simulink model "q8"  (R2019a)
settings: Solver=VariableStepAuto  StartTime=0.0  StopTime=2  RelTol=1e-3
libraries: simulink x4
settings Model: Creator=ADMIN  LastModifiedBy=ADMIN

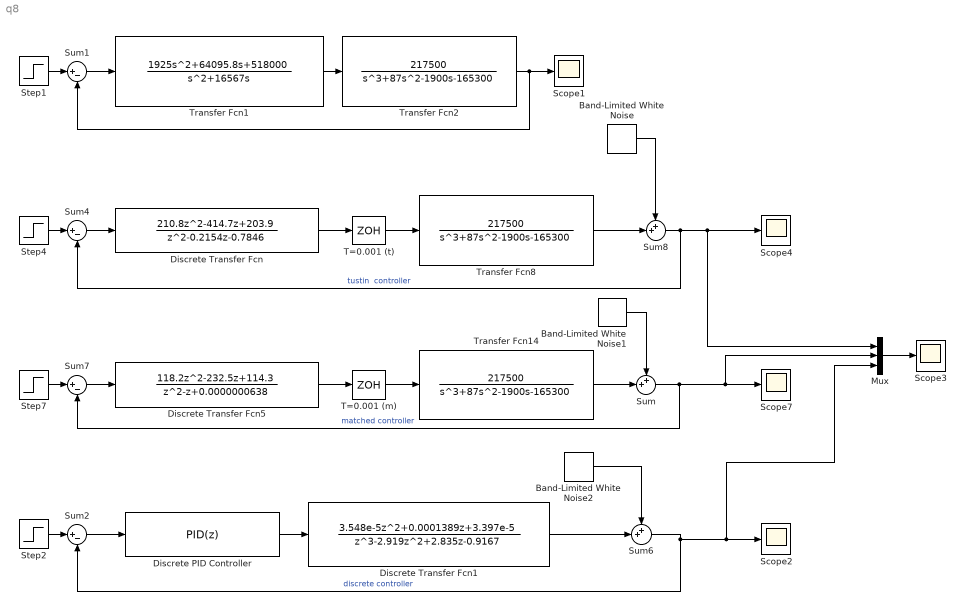
== system q8 ==
  Band-Limited White Noise : simulink/Sources/Band-Limited White Noise  Cov=[0.000001]  Ts=0.001  seed=[23341]
  Band-Limited White Noise1 : simulink/Sources/Band-Limited White Noise  Cov=[0.000001]  Ts=0.001  seed=[23341]
  Band-Limited White Noise2 : simulink/Sources/Band-Limited White Noise  Cov=[0.000001]  Ts=0.001  seed=[23341]
  Discrete Transfer Fcn : DiscreteTransferFcn  Numerator=[210.8 -414.7 203.9]  Denominator=[1 -0.2154 -0.7846]  SampleTime=0.001
  Discrete Transfer Fcn1 : DiscreteTransferFcn  Numerator=[3.548e-5 0.0001389 3.397e-5]  Denominator=[1 -2.919 2.835 -0.9167]  SampleTime=0.001
  Discrete Transfer Fcn5 : DiscreteTransferFcn  Numerator=[118.2 -232.5 114.3]  Denominator=[1 -1 0.0000000638]  SampleTime=0.001
  Discrete PID Controller : simulink/Continuous/PID Controller  Controller=PID  Form=Parallel  TimeDomain=Discrete-time  SampleTime=0.001  IntegratorMethod=Forward Euler  FilterMethod=Forward Euler  ControllerParametersSource=internal  P=6.6884073410927  I=14.7898813797399  D=0.670564929569024  UseFilter=on  N=1911.82684007629  TunerSelectOption=Transfer Function Based (PID Tuner App)  InitialConditionSource=internal  InitialConditionForIntegrator=0  InitialConditionForFilter=0  DifferentiatorICPrevScaledInput=0  ExternalReset=none  TrackingMode=off  Kt=1  LimitOutput=off  UpperSaturationLimit=inf  LowerSaturationLimit=-inf  LinearizeAsGain=off  AntiWindupMode=none  Kb=1  POutMin=[]  POutMax=[]  IOutMin=[]  IOutMax=[]  DOutMin=[]  DOutMax=[]  NOutMin=[]  NOutMax=[]  SumOutMin=[]  SumOutMax=[]  SaturationOutMin=[]  SaturationOutMax=[]  PParamMin=[]  PParamMax=[]  IParamMin=[]  IParamMax=[]  DParamMin=[]  DParamMax=[]  NParamMin=[]  NParamMax=[]  KbParamMin=[]  KbParamMax=[]  KtParamMin=[]  KtParamMax=[]  KbOutMin=[]  KbOutMax=[]  KtOutMin=[]  KtOutMax=[]  IntegratorOutMin=[]  IntegratorOutMax=[]  FilterOutMin=[]  FilterOutMax=[]  SumI1OutMin=[]  SumI1OutMax=[]  SumI2OutMin=[]  SumI2OutMax=[]  SumI3OutMin=[]  SumI3OutMax=[]  SumI4OutMin=[]  SumI4OutMax=[]  SumDOutMin=[]  SumDOutMax=[]  DifferentiatorOutMin=[]  DifferentiatorOutMax=[]  FilterDiffOutCoefMin=[]  FilterDiffOutCoefMax=[]  ReciprocalOutMin=[]  ReciprocalOutMax=[]  SumDenOutMin=[]  SumDenOutMax=[]  SumNumOutMin=[]  SumNumOutMax=[]  DivideOutMin=[]  DivideOutMax=[]  IntegratorContinuousStateAttributes=''  IntegratorStateMustResolveToSignalObject=off  IntegratorRTWStateStorageClass=Auto  FilterContinuousStateAttributes=''  FilterStateMustResolveToSignalObject=off  FilterRTWStateStorageClass=Auto  ParallelPVariant=InternalParameters  IdealPVariant=Disabled  IVariant=InternalParameters  DVariant=InternalParameters  IntegratorVariant=Discrete  SatVariant=Disabled  AWVariant=Passthrough  PCopyVariant=Disabled  TRVariant=Disabled  FdbkBlocksVariant=Forward  IdealPFdbkVariant=Disabled  SatFdbkVariant=Disabled  DerivativeFilterVariant=ForwardEulerFilter  NVariant=InternalParameters  NCopyVariant=Disabled  FilterICVariant=InternalICsFilter  IntegratorICVariant=InternalICs  ExternalResetVariant=Disabled  TRSumVariant=Passthrough  SumFdbkVariant=Disabled  SumVariant=Sum_PID
  Mux : Mux  Inputs=3
  Scope{1..4,7} (5 alike) : Scope
  Step1 : Step  Time=0  SampleTime=0
  Step2 : Step  Time=0  SampleTime=0.001
  Step4 : Step  Time=0  SampleTime=0
  Step7 : Step  Time=0  SampleTime=0
  Sum : Sum  Inputs=++|
  Sum{1..2,4,7} (4 alike) : Sum  Inputs=|+-
  Sum6 : Sum  Inputs=++|
  Sum8 : Sum  Inputs=++|
  T=0.001 (m) : ZeroOrderHold  SampleTime=0.001
  T=0.001 (t) : ZeroOrderHold  SampleTime=0.001
  Transfer Fcn1 : TransferFcn  Numerator=[1925 64095.8 518000]  Denominator=[1 16567 0]
  Transfer Fcn14 : TransferFcn  Numerator=[217500]  Denominator=[1 87 -1900 -165300]
  Transfer Fcn2 : TransferFcn  Numerator=[217500]  Denominator=[1 87 -1900 -165300]
  Transfer Fcn8 : TransferFcn  Numerator=[217500]  Denominator=[1 87 -1900 -165300]
  wires:
  Discrete Transfer Fcn/1 -> T=0.001 (t)/1
  Step4/1 -> Sum4/1
  Sum4/1 -> Discrete Transfer Fcn/1
  T=0.001 (t)/1 -> Transfer Fcn8/1
  Discrete Transfer Fcn5/1 -> T=0.001 (m)/1
  T=0.001 (m)/1 -> Transfer Fcn14/1
  Step7/1 -> Sum7/1
  Sum7/1 -> Discrete Transfer Fcn5/1
  Sum1/1 -> Transfer Fcn1/1
  Transfer Fcn2/1 -> Sum1/2, Scope1/1
  Step1/1 -> Sum1/1
  Transfer Fcn1/1 -> Transfer Fcn2/1
  Step2/1 -> Sum2/1
  Discrete PID Controller/1 -> Discrete Transfer Fcn1/1
  Sum2/1 -> Discrete PID Controller/1
  Sum/1 -> Mux/2, Scope7/1, Sum7/2  "matched controller"
  Transfer Fcn14/1 -> Sum/2
  Discrete Transfer Fcn1/1 -> Sum6/2
  Sum6/1 -> Sum2/2, Mux/3, Scope2/1  "discrete controller"
  Transfer Fcn8/1 -> Sum8/2
  Sum8/1 -> Sum4/2, Mux/1, Scope4/1  "tustin  controller"
  Band-Limited White Noise/1 -> Sum8/1
  Band-Limited White Noise1/1 -> Sum/1
  Band-Limited White Noise2/1 -> Sum6/1
  Mux/1 -> Scope3/1
